simulink model "SINGLE_INV_MPC"  (R2020b)
settings: Solver=ode23tb  StartTime=0.0  StopTime=5  RelTol=1e-3
model workspace (MAT data in the model file):
  Ts = Simulink.Parameter
  Ts.Value = 5e-06
  Ts.DataType = 'auto'
  Ts.Dimensions = [1 1]
  secondary_on = Simulink.Parameter
  secondary_on.DataType = 'auto'
  secondary_on.Dimensions = [0 0]
values from neighbouring files (symbols this model uses):
  C_f = 50e-6    (= 5e-05)    [Four_DG_MG_PrimaryOnlyScript.m]    (also in MPC_MG_script.m; MPC_MG_script_raw_dmpc.m; MPC_MG_secondary_script.m; MPG_MG_July.m)
  f_c = 5000    [Four_DG_MG_PrimaryOnlyScript.m]    (also in MPC_MG_script.m = 40000; MPC_MG_script_raw_dmpc.m = 40000; MPC_MG_secondary_script.m = 40000; MPG_MG_July.m = 50000)
  kL = 1e-5    (= 1e-05)    [Four_DG_MG_PrimaryOnlyScript.m]    (also in MPC_MG_script.m = 1e-08; MPC_MG_script_raw_dmpc.m = 1e-08; MPC_MG_secondary_script.m = 1e-07; MPG_MG_July.m = 1e-07)
  L_f = 1.35e-3    (= 0.00135)    [Four_DG_MG_PrimaryOnlyScript.m]    (also in MPC_MG_script.m; MPC_MG_script_raw_dmpc.m; MPC_MG_secondary_script.m; MPG_MG_July.m)
  L_in1 = 0.35e-3    (= 0.00035)    [Four_DG_MG_PrimaryOnlyScript.m]    (also in MPC_MG_script.m; MPC_MG_script_raw_dmpc.m; MPC_MG_secondary_script.m; MPG_MG_July.m)
  LD_ref1 = 800e-6    (= 0.0008)    [Four_DG_MG_PrimaryOnlyScript.m]    (also in MPC_MG_script.m = 0.0003; MPC_MG_script_raw_dmpc.m = 0.0003; MPC_MG_secondary_script.m = 0.0001; MPG_MG_July.m = 0.0004)
  lo_co = 0.2    [Four_DG_MG_PrimaryOnlyScript.m]    (also in MPC_MG_script.m = 0.05; MPC_MG_script_raw_dmpc.m; MPC_MG_secondary_script.m = 0.08; MPG_MG_July.m = 0.15)
  m_p1 = 9.4e-5/droopDivide    (= 9.4e-05)    [Four_DG_MG_PrimaryOnlyScript.m]    (also in MPC_MG_script.m; MPC_MG_script_raw_dmpc.m; MPC_MG_secondary_script.m; MPG_MG_July.m)
  n_q1 = 1.3e-3/droopDivide2    (= 0.00013)    [Four_DG_MG_PrimaryOnlyScript.m]    (also in MPC_MG_script.m; MPC_MG_script_raw_dmpc.m; MPC_MG_secondary_script.m; MPG_MG_July.m)
  R_f = 0.1    [Four_DG_MG_PrimaryOnlyScript.m]    (also in MPC_MG_script.m; MPC_MG_script_raw_dmpc.m; MPC_MG_secondary_script.m; MPG_MG_July.m)
  R_in1 = 0.03    [Four_DG_MG_PrimaryOnlyScript.m]    (also in MPC_MG_script.m; MPC_MG_script_raw_dmpc.m; MPC_MG_secondary_script.m; MPG_MG_July.m)
  Ts = 10e-6    (= 1e-05)    [Four_DG_MG_PrimaryOnlyScript.m]    (also in MPC_MG_script.m; MPC_MG_script_raw_dmpc.m; MPC_MG_secondary_script.m; MPG_MG_July.m)
  V_nom = 220*sqrt(2)    [Four_DG_MG_PrimaryOnlyScript.m]    (also in MPC_MG_script.m; MPC_MG_script_raw_dmpc.m; MPC_MG_secondary_script.m; MPG_MG_July.m)
  Vdc = 600    [Four_DG_MG_PrimaryOnlyScript.m]    (also in MPC_MG_script.m; MPC_MG_script_raw_dmpc.m; MPC_MG_secondary_script.m; MPG_MG_July.m)
  w_c_high = 2*pi*50    (= 314.159265359)    [Four_DG_MG_PrimaryOnlyScript.m]    (also in MPC_MG_script.m; MPC_MG_script_raw_dmpc.m; MPC_MG_secondary_script.m; MPG_MG_July.m)
  w_nom = 2*pi*50    (= 314.159265359)    [Four_DG_MG_PrimaryOnlyScript.m]    (also in MPC_MG_script.m; MPC_MG_script_raw_dmpc.m; MPC_MG_secondary_script.m; MPG_MG_July.m)
undefined symbols (not defined in the file or in its folder): i
libraries: powerlib x11, powerlib_meascontrol x7, eeGeneralControl x2, dspswit3 x1
settings Model: SimulationMode=accelerator  Creator=Linh  LastModifiedBy=Linh
settings DataIOCC: ReturnWorkspaceOutputs=off

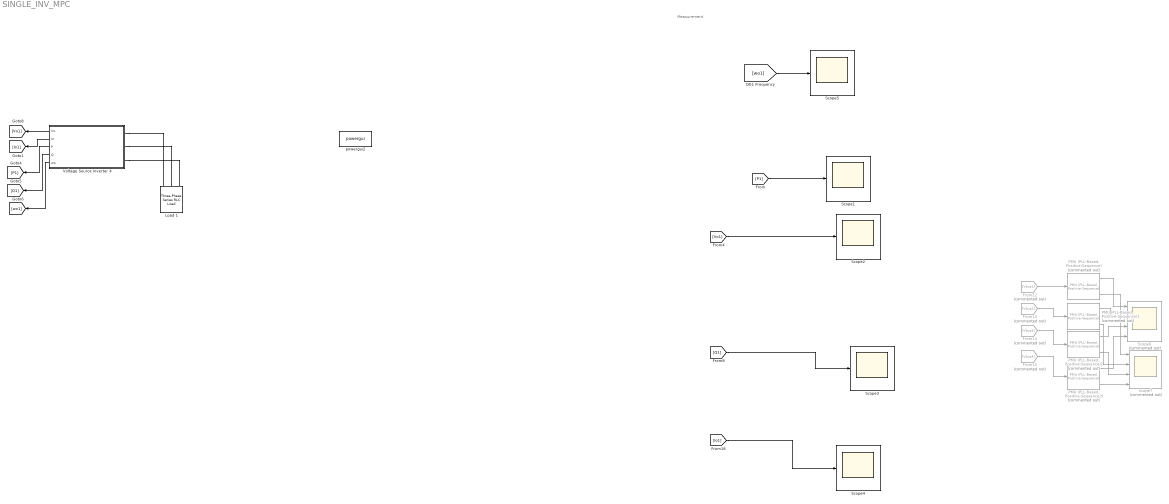
== system SINGLE_INV_MPC ==
  note: Measurement
  From12 : From  Commented=on  GotoTag=Vbus1  TagVisibility=global
  From13 : From  Commented=on  GotoTag=Vbus2  TagVisibility=global
  From14 : From  Commented=on  GotoTag=Vbus3  TagVisibility=global
  From15 : From  Commented=on  GotoTag=Vbus4  TagVisibility=global
  Load 1 : powerlib/Elements/Three-Phase Series RLC Load  LConnTagsString=A|B|C  Configuration=Y (grounded)  NominalVoltage=220*sqrt(3)  Vabc=[1e3 1e3 1e3]  Vabcp=[1e3 1e3 1e3]  NominalFrequency=50  UnbalancedPower=off  ActivePower=12000*3  InductivePower=12000*3  CapacitivePower=0  Pabc=[10e3 9e3 11e3]  QLabc=[100 90 110]  QCabc=[100 90 110]  Pabcp=[10e3 9e3 11e3]  QLabcp=[100 90 110]  QCabcp=[100 90 110]  Measurements=Branch voltages and currents  LoadType=constant Z
  PMU (PLL-Based, Positive-Sequence){,1..3} (4 alike) : powerlib_meascontrol/Measurements/PMU (PLL-Based, Positive-Sequence)  Commented=on  nominalFrequency=50  samplingRate=64  reportingFactor=5
      settings: SourceProductBaseCode=PS
  Scope{1..5} (5 alike) : Scope
  Scope6 : Scope  Commented=on  NumInputPorts=4
  Scope7 : Scope  Commented=on  NumInputPorts=4
  Voltage Source Inverter 4 : Subsystem  mask{w_nom=w_nom, V_nom=V_nom, modT=1/f_c, m_p=m_p1, n_q=n_q1, LD_ref=LD_ref1, k_LD=kL, w_c_high=[1 w_c_high], R_f=R_f, L_f=L_f, C_f=C_f, R_in=R_in1, L_in=L_in1}
      mask prompts: w_nom "Nominal frequency (radian)"; V_nom "Nominal voltage"; modT "Sampling Time"; m_p "P-w gain"; n_q "Q-V gain"; LD_ref "Reference virtual impedance (H)"; k_LD "Virtual impedance Q gain"; w_c_high "High-pass filter denominator:"; R_f "Inductor resistance:"; L_f "Filter inductance"; C_f "Filter capacitance"; R_in "Resistance coupling"; L_in "Inductance coupling"
      mask TypeOptions w_nom: w_nom/Value
      mask TypeOptions V_nom: V_nom/Value
      mask TypeOptions modT:
      | Model Predictive Control
      | /Ts
      mask TypeOptions m_p: Droop for secondary control2/Gain5/Gain
      mask TypeOptions n_q: Droop for secondary control2/Gain4/Gain
      mask TypeOptions LD_ref: LD_ref/Value
      mask TypeOptions k_LD: k_LD/Gain
      mask TypeOptions w_c_high: High-Pass Filter/Denominator
      mask TypeOptions R_f:
      | Three-Phase
      | Series RLC Branch/Resistance
      mask TypeOptions L_f:
      | Three-Phase
      | Series RLC Branch/Inductance
      mask TypeOptions C_f:
      | Three-Phase
      | Series RLC Branch2/Capacitance
      mask TypeOptions R_in:
      | Three-Phase
      | Series RLC Branch1/Resistance
      mask TypeOptions L_in:
      | Three-Phase
      | Series RLC Branch1/Inductance
      mask DialogControl ParameterGroupVar Prompt: Microgrid-wide values
      mask DialogControl Container5 Prompt: Droop value
      mask DialogControl Container8 Prompt: Filter
  powergui2 : powerlib/powergui  Priority=1  SimulationMode=Discrete  SampleTime=Ts  frequency=60  Iterations=50  frequencyindice=0  Pbase=100e6  ErrMax=1e-4  UnitsV=kV  UnitsW=MW  buscounter=0  FunctionMessages=off  echomessages=off  EnableUseOfTLC=off  CurrentSourceSwitches=off  DisableSnubberDevices=off  DisableRonSwitches=off  DisableVfSwitches=off  DisplayEquations=off  AutomaticDiscreteSolvers=off  SolverType=Tustin/Backward Euler (TBE)  Interpol=off  ExternalGateDelay=off  methode=off  Ts=100  x0status=blocks  SPID=on  SwTol=0  HookPort=off  NonlinearTolerance=1e-4  nMaxIteration=100  ContinueOnMaxIteration=off  RestoreLinks=warning  ResistiveCurrentMeasurement=off  Frange=[0:2:500]  Ylog=off  Xlog=on  ShowGrid=off  save=off  variable=ZData  structure=Voltage  ZoomFFT=off  StartTime=0.015  cycles=10  DisplayStyle=1  fundamental=50  FreqAxis=on  MaxFrequency=1000  frequencyindicesteady=1  RmsSteady=1  display=off
  wires:
  Voltage Source Inverter 4/1(Vo) -> [Vo1]
  Voltage Source Inverter 4/2(Io) -> [Io1]
  Voltage Source Inverter 4/3(P) -> [P1]
  Voltage Source Inverter 4/4(Q) -> [Q1]
  Voltage Source Inverter 4/5(wo) -> [wo1]
  "PMU (PLL-Based, Positive-Sequence)1"/3 -> Scope7/2
  From12/1 -> "PMU (PLL-Based, Positive-Sequence)"/1
  [Q1] -> Scope3/1
  "PMU (PLL-Based, Positive-Sequence)3"/1 -> Scope6/4
  "PMU (PLL-Based, Positive-Sequence)2"/3 -> Scope7/3
  "PMU (PLL-Based, Positive-Sequence)2"/1 -> Scope6/3
  From14/1 -> "PMU (PLL-Based, Positive-Sequence)2"/1
  [P1] -> Scope1/1
  "PMU (PLL-Based, Positive-Sequence)3"/3 -> Scope7/4
  "PMU (PLL-Based, Positive-Sequence)"/1 -> Scope6/1
  "PMU (PLL-Based, Positive-Sequence)"/3 -> Scope7/1
  "PMU (PLL-Based, Positive-Sequence)1"/1 -> Scope6/2
  From13/1 -> "PMU (PLL-Based, Positive-Sequence)1"/1
  [Vo1] -> Scope2/1
  [wo1] -> Scope5/1
  From15/1 -> "PMU (PLL-Based, Positive-Sequence)3"/1
  [Io1] -> Scope4/1
  connections:
  Voltage Source Inverter 4/LConn3 -- Load 1/LConn3
  Voltage Source Inverter 4/LConn2 -- Load 1/LConn2
  Voltage Source Inverter 4/LConn1 -- Load 1/LConn1

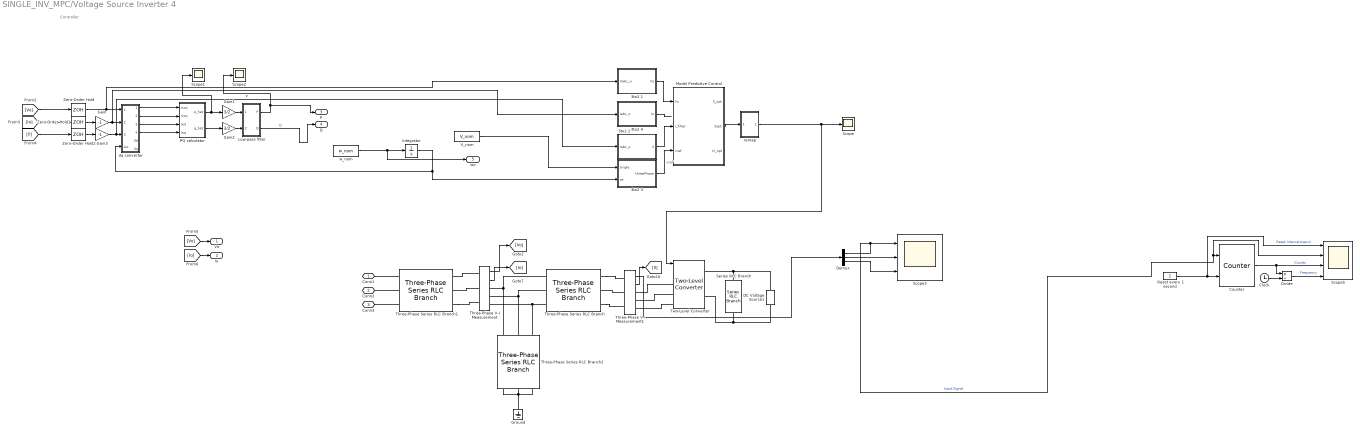
== system SINGLE_INV_MPC/Voltage Source Inverter 4 ==
  note: Controller
  3to2 1 : Subsystem
  3to2 2 : Subsystem
  3to2 3 : Subsystem
  3to2 4 : Subsystem
  Clock : Clock
  Counter : dspswit3/Counter  Direction=Up  CountEvent=Rising edge  CounterSize=User defined  MaxCount=15e3  InitialCount=0  Output=Count  HitValue=1  ResetInput=on  SamplesPerFrame=1  Ts=1  CntDtype=double  HitDtype=Logical
  DC Voltage Source1 : powerlib/Electrical Sources/DC Voltage Source  Amplitude=Vdc  Measurements=None
  Demux : Demux  Outputs=3
  Divide : Product  Inputs=*/
  Gain : Gain  Gain=-1
  Gain1 : Gain  Gain=3/2
  Gain2 : Gain  Gain=3/2
  Gain3 : Gain  Gain=-1
  Ground : powerlib/Elements/Ground  LConnTagsString=a
  Integrator : Integrator  WrapState=on  WrappedStateUpperValue=2*pi  WrappedStateLowerValue=0
  Low-pass filter : Subsystem
  "Model Predictive Control " : MATLAB Function  TreatAsAtomicUnit=on  mask{Ts=modT, Cfilter=C_f, Lfilter=L_f, Vdc=Vdc}
      mask prompts: Ts "Sampling Time"; Cfilter "Filter Capacitor"; Lfilter "Filter Inductance"; Vdc "Input DC Voltage"
  PQ calculator : Subsystem
  Reset every 1 second : Constant
  Scope : Scope
  Scope1 : Scope
  Scope2 : Scope
  Scope3 : Scope  NumInputPorts=3
  Scope5 : Scope  NumInputPorts=4
  Series RLC Branch : powerlib/Elements/Series RLC Branch  LConnTagsString=__new0  RConnTagsString=__new0  BranchType=RC  Resistance=30  Inductance=1e-3  SetiL0=off  InitialCurrent=0  Capacitance=80e-6  Setx0=off  InitialVoltage=0  Measurements=None
  Three-Phase Series RLC Branch : powerlib/Elements/Three-Phase Series RLC Branch  LConnTagsString=A|B|C  RConnTagsString=A|B|C  BranchType=RL  Resistance=R_f  Inductance=L_f  Capacitance=1e-6  Measurements=None
  Three-Phase Series RLC Branch1 : powerlib/Elements/Three-Phase Series RLC Branch  LConnTagsString=A|B|C  RConnTagsString=A|B|C  BranchType=RL  Resistance=R_in  Inductance=L_in  Capacitance=1e-6  Measurements=None
  Three-Phase Series RLC Branch2 : powerlib/Elements/Three-Phase Series RLC Branch  LConnTagsString=A|B|C  RConnTagsString=A|B|C  BranchType=C  Resistance=R_f  Inductance=1e-3  Capacitance=C_f  Measurements=None
  Three-Phase V-I Measurement : powerlib/Measurements/Three-Phase V-I Measurement  VoltageMeasurement=phase-to-ground  SetLabelV=off  LabelV=Vo1  Vpu=off  VpuLL=off  CurrentMeasurement=yes  SetLabelI=off  LabelI=Io1  Ipu=off  Pbase=100e6  Vbase=500e3  OutputType=Complex  PhasorSimulation=off  PSBequivalent=0
  Three-Phase V-I Measurement1 : powerlib/Measurements/Three-Phase V-I Measurement  VoltageMeasurement=phase-to-ground  SetLabelV=off  LabelV=Vl2  Vpu=off  VpuLL=off  CurrentMeasurement=yes  SetLabelI=off  LabelI=Il2  Ipu=off  Pbase=100e6  Vbase=500e3  OutputType=Complex  PhasorSimulation=off  PSBequivalent=0
  Two-Level Converter : powerlib/Power Electronics/Two-Level Converter  ModelType=Switching devices  Ron=1e-3  Rs=1e6  Cs=inf  Vforward=[0,0]  Ron_Diode=1e-3  Rs_Diode=1e6  Cs_Diode=inf  Vf_Diode=1e-3  Rs_CurrentSource=inf
      settings: SourceProductBaseCode=PS
  V_nom : Constant  Value=V_nom
  Zero-Order Hold : ZeroOrderHold  SampleTime=modT
  Zero-Order Hold1 : ZeroOrderHold  SampleTime=modT
  Zero-Order Hold2 : ZeroOrderHold  SampleTime=modT
  dq converter : Subsystem
  remap : Subsystem
  w_nom : Constant  Value=w_nom
  Conn1 : PMIOPort  Side=Left
  Conn2 : PMIOPort  Port=2  Side=Left
  Conn3 : PMIOPort  Port=3  Side=Left
  Vo : Outport
  Io : Outport  Port=2
  P : Outport  Port=3
  Q : Outport  Port=4
  wo : Outport  Port=5
  wires:
  Gain/1 -> 3to2 4/1("Iabc_o "), dq converter/2(Iodq)
  Integrator/1 -> dq converter/4(wo), 3to2 3/2("wt ")
  Low-pass filter/2(Q) -> Q/1  "Q"
  Gain2/1 -> Low-pass filter/2(q_hat)
  Low-pass filter/1(P) -> Scope2/1, P/1  "P"
  PQ calculator/2(q_hat) -> Gain2/1
  Gain1/1 -> Low-pass filter/1(p_hat)
  dq converter/2(Voq) -> PQ calculator/2(Voq)
  dq converter/3(Iod) -> PQ calculator/3(Iod)
  dq converter/4(Ioq) -> PQ calculator/4(Ioq)
  [Il] -> Zero-Order Hold2/1
  PQ calculator/1(p_hat) -> Scope1/1, Gain1/1
  [Io] -> Zero-Order Hold1/1
  dq converter/1(Vod) -> PQ calculator/1(Vod)
  [Vo] -> Vo/1
  [Io] -> Io/1
  Three-Phase V-I Measurement/1 -> [Vo]
  Three-Phase V-I Measurement/2 -> [Io]
  Three-Phase V-I Measurement1/2 -> [Il]
  3to2 1/1(Vo) -> "Model Predictive Control "/1(Vc)
  3to2 3/1(threePhase) -> "Model Predictive Control "/3(vref)  "vref"
  3to2 2/1(Il) -> "Model Predictive Control "/2(i_filter)
  [Vo] -> Zero-Order Hold/1
  "Model Predictive Control "/2(Sopt) -> remap/1(In1)
  Gain3/1 -> 3to2 2/1("Iabc_o "), dq converter/3(Ildq)
  remap/1(Out1) -> Scope/1, Two-Level Converter/1
  Zero-Order Hold/1 -> 3to2 1/1("Vabc_o "), dq converter/1(Vodq)
  Zero-Order Hold1/1 -> Gain/1
  Zero-Order Hold2/1 -> Gain3/1
  w_nom/1 -> wo/1, Integrator/1
  V_nom/1 -> 3to2 3/1("single ")
  Demux/2 -> Scope3/2
  Demux/3 -> Scope3/3
  Three-Phase V-I Measurement1/1 -> Demux/1
  3to2 4/1(Io) -> ?
  Divide/1 -> Scope5/4  "Frequency"
  Reset every 1 second/1 -> Scope5/1, Counter/2  "Reset Intervals(secs)"
  Clock/1 -> Divide/2
  Counter/1 -> Scope5/3, Divide/1  "Counts"
  Demux/1 -> Scope3/1, Counter/1, Scope5/2  "Input Signal"
  connections:
  Three-Phase Series RLC Branch2/LConn1 -- Three-Phase V-I Measurement/RConn1 -- Three-Phase Series RLC Branch/LConn1
  Two-Level Converter/RConn1 -- DC Voltage Source1/RConn1 -- Series RLC Branch/LConn1
  Three-Phase Series RLC Branch2/RConn3 -- Three-Phase Series RLC Branch2/RConn1 -- Three-Phase Series RLC Branch2/RConn2 -- Ground/LConn1
  Three-Phase Series RLC Branch2/LConn3 -- Three-Phase Series RLC Branch/LConn3 -- Three-Phase V-I Measurement/RConn3
  Two-Level Converter/RConn2 -- Series RLC Branch/RConn1 -- DC Voltage Source1/LConn1
  Three-Phase Series RLC Branch/LConn2 -- Three-Phase V-I Measurement/RConn2 -- Three-Phase Series RLC Branch2/LConn2
  Two-Level Converter/LConn1 -- Three-Phase V-I Measurement1/RConn1
  Three-Phase V-I Measurement1/LConn2 -- Three-Phase Series RLC Branch/RConn2
  Two-Level Converter/LConn2 -- Three-Phase V-I Measurement1/RConn2
  Three-Phase Series RLC Branch1/LConn2 -- Conn2/RConn1
  Two-Level Converter/LConn3 -- Three-Phase V-I Measurement1/RConn3
  Three-Phase Series RLC Branch/RConn1 -- Three-Phase V-I Measurement1/LConn1
  Three-Phase Series RLC Branch1/LConn3 -- Conn3/RConn1
  Three-Phase V-I Measurement/LConn1 -- Three-Phase Series RLC Branch1/RConn1
  Three-Phase Series RLC Branch1/LConn1 -- Conn1/RConn1
  Three-Phase V-I Measurement/LConn2 -- Three-Phase Series RLC Branch1/RConn2
  Three-Phase Series RLC Branch1/RConn3 -- Three-Phase V-I Measurement/LConn3
  Three-Phase Series RLC Branch/RConn3 -- Three-Phase V-I Measurement1/LConn3

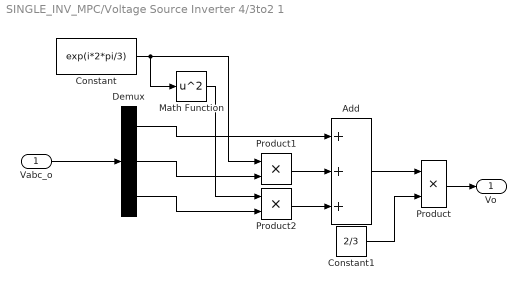
== system SINGLE_INV_MPC/Voltage Source Inverter 4/3to2 1 ==
  "Vabc_o " : Inport
  Add : Sum  Inputs=+++
  Constant : Constant  Value=exp(i*2*pi/3)
  Constant1 : Constant  Value=2/3
  Demux : Demux  Outputs=3
  Math Function : Math  Operator=square  SignedPower=on  SaturateOnIntegerOverflow=on
  Product : Product  RndMeth=Zero
  Product1 : Product  RndMeth=Zero
  Product2 : Product  RndMeth=Zero
  Vo : Outport  VectorParamsAs1DForOutWhenUnconnected=off
  wires:
  Add/1 -> Product/1
  Demux/1 -> Add/1
  Constant1/1 -> Product/2
  Product1/1 -> Add/2
  Constant/1 -> Product1/1, Math Function/1
  Demux/2 -> Product1/2
  Math Function/1 -> Product2/1
  Demux/3 -> Product2/2
  Product2/1 -> Add/3
  Product/1 -> Vo/1
  "Vabc_o "/1 -> Demux/1

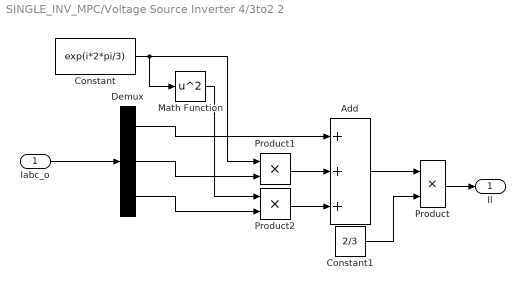
== system SINGLE_INV_MPC/Voltage Source Inverter 4/3to2 2 ==
  "Iabc_o " : Inport
  Add : Sum  Inputs=+++
  Constant : Constant  Value=exp(i*2*pi/3)
  Constant1 : Constant  Value=2/3
  Demux : Demux  Outputs=3
  Math Function : Math  Operator=square  SignedPower=on  SaturateOnIntegerOverflow=on
  Product : Product  RndMeth=Zero
  Product1 : Product  RndMeth=Zero
  Product2 : Product  RndMeth=Zero
  Il : Outport  VectorParamsAs1DForOutWhenUnconnected=off
  wires:
  Add/1 -> Product/1
  Demux/1 -> Add/1
  Constant1/1 -> Product/2
  Product1/1 -> Add/2
  Constant/1 -> Product1/1, Math Function/1
  Demux/2 -> Product1/2
  Math Function/1 -> Product2/1
  Demux/3 -> Product2/2
  Product2/1 -> Add/3
  Product/1 -> Il/1
  "Iabc_o "/1 -> Demux/1

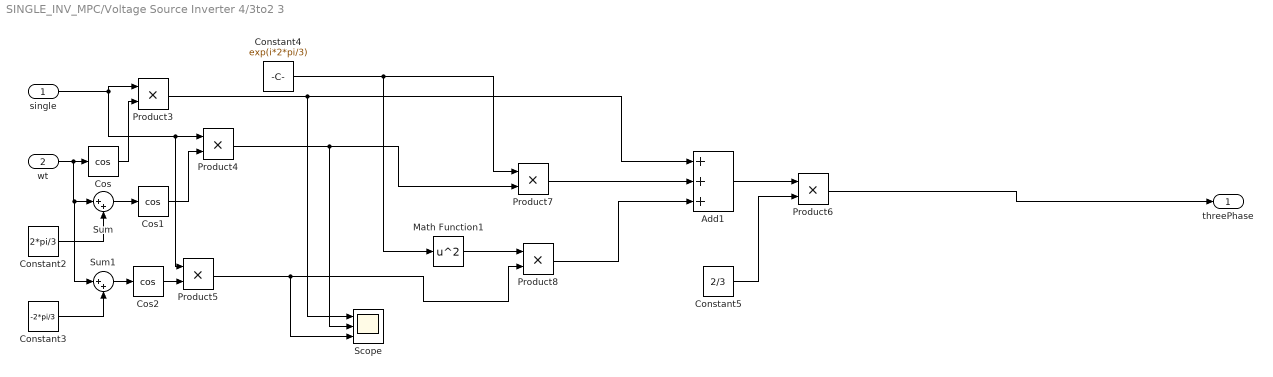
== system SINGLE_INV_MPC/Voltage Source Inverter 4/3to2 3 ==
  "single " : Inport
  "wt " : Inport  Port=2
  Add1 : Sum  Inputs=+++
  Constant2 : Constant  Value=2*pi/3
  Constant3 : Constant  Value=-2*pi/3
  Constant4 : Constant  Value=exp(i*2*pi/3)
  Constant5 : Constant  Value=2/3
  Cos : Trigonometry  Operator=cos
  Cos1 : Trigonometry  Operator=cos
  Cos2 : Trigonometry  Operator=cos
  Math Function1 : Math  Operator=square  SignedPower=on  SaturateOnIntegerOverflow=on
  Product{3..8} (6 alike) : Product  RndMeth=Zero
  Scope : Scope  NumInputPorts=3
  Sum : Sum  Inputs=|++
  Sum1 : Sum  Inputs=|++
  threePhase : Outport  VectorParamsAs1DForOutWhenUnconnected=off
  wires:
  "single "/1 -> Product5/1, Product4/1, Product3/1
  Cos/1 -> Product3/2
  Constant2/1 -> Sum/2
  Sum/1 -> Cos1/1
  Cos1/1 -> Product4/2
  "wt "/1 -> Sum1/1, Sum/1, Cos/1
  Constant3/1 -> Sum1/2
  Sum1/1 -> Cos2/1
  Cos2/1 -> Product5/2
  Constant4/1 -> Product7/1, Math Function1/1
  Product7/1 -> Add1/2
  Add1/1 -> Product6/1
  Product8/1 -> Add1/3
  Product5/1 -> Scope/3, Product8/2
  Product6/1 -> threePhase/1
  Product3/1 -> Scope/1, Add1/1
  Constant5/1 -> Product6/2
  Product4/1 -> Scope/2, Product7/2
  Math Function1/1 -> Product8/1

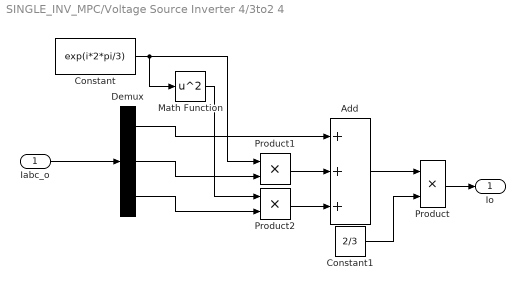
== system SINGLE_INV_MPC/Voltage Source Inverter 4/3to2 4 ==
  "Iabc_o " : Inport
  Add : Sum  Inputs=+++
  Constant : Constant  Value=exp(i*2*pi/3)
  Constant1 : Constant  Value=2/3
  Demux : Demux  Outputs=3
  Math Function : Math  Operator=square  SignedPower=on  SaturateOnIntegerOverflow=on
  Product : Product  RndMeth=Zero
  Product1 : Product  RndMeth=Zero
  Product2 : Product  RndMeth=Zero
  Io : Outport  VectorParamsAs1DForOutWhenUnconnected=off
  wires:
  Add/1 -> Product/1
  Demux/1 -> Add/1
  Constant1/1 -> Product/2
  Product1/1 -> Add/2
  Constant/1 -> Product1/1, Math Function/1
  Demux/2 -> Product1/2
  Math Function/1 -> Product2/1
  Demux/3 -> Product2/2
  Product2/1 -> Add/3
  Product/1 -> Io/1
  "Iabc_o "/1 -> Demux/1

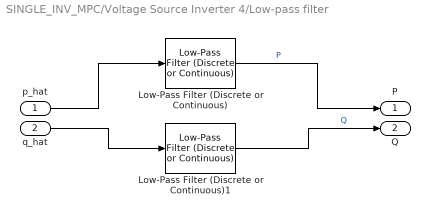
== system SINGLE_INV_MPC/Voltage Source Inverter 4/Low-pass filter ==
  p_hat : Inport
  q_hat : Inport  Port=2
  Low-Pass Filter (Discrete or Continuous) : eeGeneralControl/Low-Pass Filter (Discrete or Continuous)  K=1  T=lo_co  B=inf  A=-inf  init_option=Inherited from block input  x0=0  Ts=-1
  Low-Pass Filter (Discrete or Continuous)1 : eeGeneralControl/Low-Pass Filter (Discrete or Continuous)  K=1  T=lo_co  B=inf  A=-inf  init_option=Inherited from block input  x0=0  Ts=-1
  P : Outport
  Q : Outport  Port=2
  wires:
  q_hat/1 -> Low-Pass Filter (Discrete or Continuous)1/1
  Low-Pass Filter (Discrete or Continuous)1/1 -> Q/1  "Q"
  Low-Pass Filter (Discrete or Continuous)/1 -> P/1  "P"
  p_hat/1 -> Low-Pass Filter (Discrete or Continuous)/1

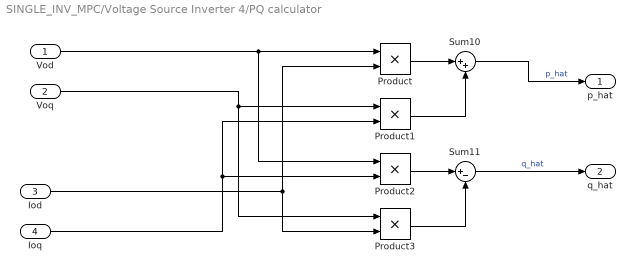
== system SINGLE_INV_MPC/Voltage Source Inverter 4/PQ calculator ==
  Vod : Inport
  Voq : Inport  Port=2
  Iod : Inport  Port=3
  Ioq : Inport  Port=4
  Product{,1..3} (4 alike) : Product
  Sum10 : Sum  Inputs=|++
  Sum11 : Sum  Inputs=|+-
  p_hat : Outport
  q_hat : Outport  Port=2
  wires:
  Product3/1 -> Sum11/2
  Product1/1 -> Sum10/2
  Voq/1 -> Product3/1, Product1/1
  Iod/1 -> Product/2, Product3/2
  Product2/1 -> Sum11/1
  Ioq/1 -> Product1/2, Product2/2
  Product/1 -> Sum10/1
  Vod/1 -> Product/1, Product2/1
  Sum11/1 -> q_hat/1  "q_hat"
  Sum10/1 -> p_hat/1  "p_hat"

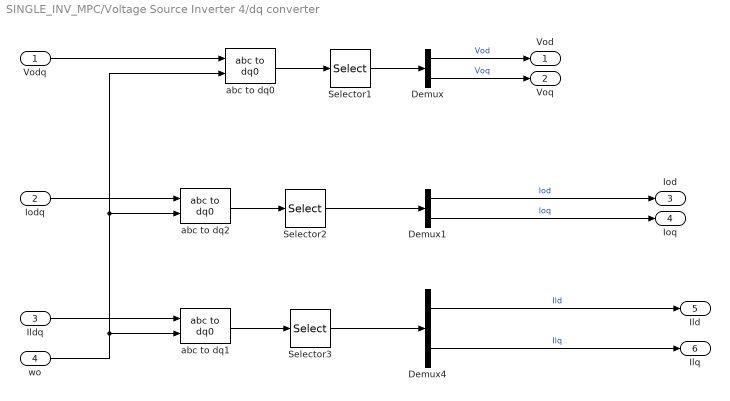
== system SINGLE_INV_MPC/Voltage Source Inverter 4/dq converter ==
  Vodq : Inport
  Iodq : Inport  Port=2
  Ildq : Inport  Port=3
  wo : Inport  Port=4
  Demux : Demux  Outputs=2
  Demux1 : Demux  Outputs=2
  Demux4 : Demux  Outputs=2
  Selector1 : Selector  InputPortWidth=3  IndexOptions=Index vector (dialog)  Indices=[1 2]  OutputSizes=1
  Selector2 : Selector  InputPortWidth=3  IndexOptions=Index vector (dialog)  Indices=[1 2]  OutputSizes=1
  Selector3 : Selector  InputPortWidth=3  IndexOptions=Index vector (dialog)  Indices=[1 2]  OutputSizes=1
  abc to dq0 : powerlib_meascontrol/Transformations/abc to dq0  Alignment=90 degrees behind phase A axis
  abc to dq1 : powerlib_meascontrol/Transformations/abc to dq0  Alignment=90 degrees behind phase A axis
  abc to dq2 : powerlib_meascontrol/Transformations/abc to dq0  Alignment=90 degrees behind phase A axis
  Vod : Outport
  Voq : Outport  Port=2
  Iod : Outport  Port=3
  Ioq : Outport  Port=4
  Ild : Outport  Port=5
  Ilq : Outport  Port=6
  wires:
  Vodq/1 -> abc to dq0/1
  Demux/1 -> Vod/1  "Vod"
  Demux1/1 -> Iod/1  "Iod"
  Selector3/1 -> Demux4/1
  Demux/2 -> Voq/1  "Voq"
  Selector1/1 -> Demux/1
  abc to dq2/1 -> Selector2/1
  abc to dq1/1 -> Selector3/1
  wo/1 -> abc to dq0/2, abc to dq2/2, abc to dq1/2
  Demux1/2 -> Ioq/1  "Ioq"
  Demux4/1 -> Ild/1  "Ild"
  abc to dq0/1 -> Selector1/1
  Selector2/1 -> Demux1/1
  Iodq/1 -> abc to dq2/1
  Ildq/1 -> abc to dq1/1
  Demux4/2 -> Ilq/1  "Ilq"

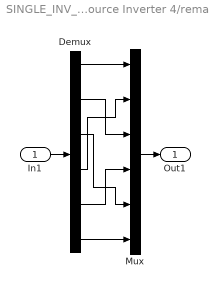
== system SINGLE_INV_MPC/Voltage Source Inverter 4/remap ==
  In1 : Inport
  Demux : Demux  Outputs=6
  Mux : Mux  Inputs=6
  Out1 : Outport
  wires:
  Demux/5 -> Mux/4
  Demux/3 -> Mux/5
  Demux/2 -> Mux/3
  Demux/4 -> Mux/2
  In1/1 -> Demux/1
  Demux/1 -> Mux/1
  Demux/6 -> Mux/6
  Mux/1 -> Out1/1

== matlab function SINGLE_INV_MPC/Voltage Source Inverter 4/Model Predictive Control  ==
  settings: updateMethod=DISCRETE  sampleTime=Ts
  data: S_opt output; Sopt output size=[1 6]; Vc input; i_filter input; vref input; Vi_opt output; Vdc parameter double size=1; modT parameter size=1; Cfilter parameter size=1; Lfilter parameter size=1
function [S_opt, Sopt, Vi_opt] = MPC(Vc, i_filter,vref,Vdc,modT,Cfilter,Lfilter)

    % In order to call "cont2dis" function
    coder.extrinsic('cont2dis');
    persistent Aq Bq Bdq Vc1 if1 Vc_old if_old x_opt g 

    % Initialize variables and get the parameters of the Discrete model based on Ts
    if isempty(x_opt), x_opt = 1; end
    if isempty(Vc1), Vc1 = 0 + 1j*0; end
    if isempty(Vc_old), Vc_old = 0 + 1j*0; end
    if isempty(if_old), if_old = 0 + 1j*0; end
    if isempty(if1), if1 = 0 + 1j*0; end
    
    if isempty(Aq) && isempty(Bq) && isempty(Bdq)
        Aq = zeros(2);     Bq = zeros(2,1);     Bdq = zeros(2,1);
        % Call "cont2dis" function
        [Aq, Bq, Bdq] = cont2dis(modT,Lfilter,Cfilter); 
    end
    
    % Intialize the cost function
    g_opt = inf;
    
    % To generate the switching states matrix
    states = [1 0 0;
              0 0 0  
              1 1 0
              0 1 0
              0 1 1
              0 0 1
              1 0 1
              1 1 1];
    a = exp(1j*(2*pi/3));
    
    % Read current measurements at sampling instant k
    ifk = i_filter;
    Vck = Vc;
    % Equation of io(k-1) = if(k-1)-(c/Ts)(vc(k)-vc(k-1)).
    io = if_old - (Cfilter/modT)*(Vck - Vc_old); 
    
    % Store the measured current for the next iteration
    if_old = ifk;
    Vc_old = Vck;
    % FOR loop to find the best switch in the next instant and its corresponding V(i)
    for k = 1:8
        s = states(k,:);
        sw = (2/3)*(s(1)+a*s(2)+a^2*s(3));
        Vi = Vdc*sw;

        % Output Voltage Prediction at instant k+1
        if1 = Aq(1,1)*ifk + Aq(1,2)*Vck + Bq(1)*Vi + Bdq(1)*io; 
        Vc1 = Aq(2,1)*ifk + Aq(2,2)*Vck + Bq(2)*Vi + Bdq(2)*io; 
        Nc = sum(abs(states(k,:)-states(x_opt,:)))^2;    
        g1 = (real(if1)-real(io)+Cfilter*2*pi*50*imag(vref))^2 + (imag(if1)-imag(io)+Cfilter*2*pi*50*real(vref))^2;
        g = (real(vref)-real(Vc1))^2+(imag(vref)-imag(Vc1))^2 + 0.1*g1;
        
        if (g < g_opt)
            x_opt = k;
            g_opt = g;
        end  
    end
    % Output switching states and its voltage vector. 
    Vi_opt = x_opt; 
    S_opt = states(x_opt,:);
    d_opt = not(S_opt);
    Sopt = [S_opt,d_opt];     
end
